simulink model "model_dyskr_z_kwantyzatorem"  (Simulink 7.5)
settings: Solver=ode45  StartTime=0.0  StopTime=5  FixedStep=0.006  MinStep=0.0006  RelTol=1e-3
undefined symbols (not defined in the file): In, J, K1, K2, Kp, Kt, lambdaN, m, Mn, psien, Rt, T, tm, Tp, Un, uz0, V, wn, Y
settings Model: Creator=Konrad  LastModifiedBy=Konrad

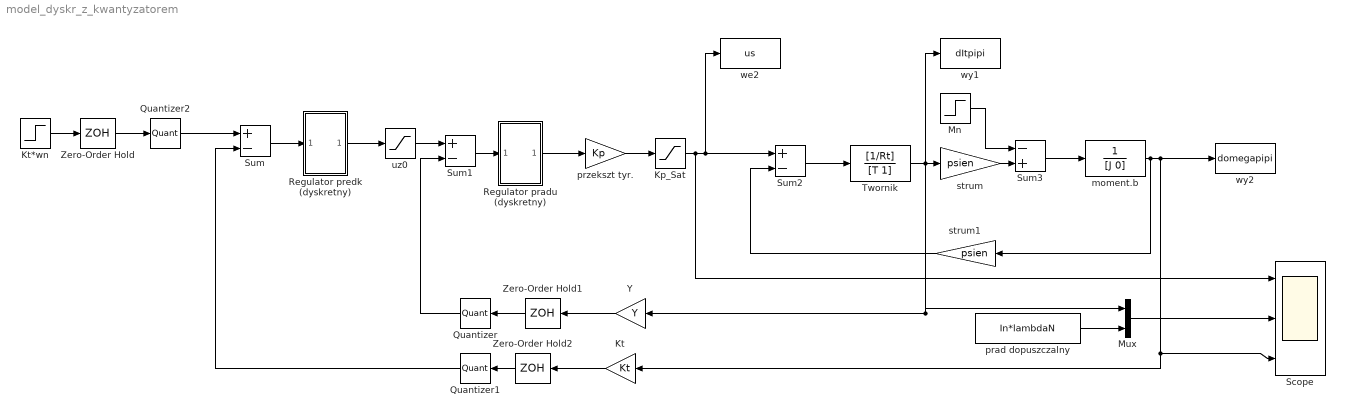
== system model_dyskr_z_kwantyzatorem ==
  Kp_Sat : Saturate  UpperLimit=1.5*Un  LowerLimit=-1.5*Un  OutDataType=fixdt(1, 16)  OutScaling=2^0
  Kt : Gain  Gain=Kt  ParameterDataType=fixdt(1, 16)  ParameterScaling=2^0  OutDataType=fixdt(1, 16)  OutScaling=2^0
  Kt*wn : Step  Time=0  After=Kt*wn  SampleTime=0
  Mn : Step  Time=tm  After=Mn  SampleTime=0
  Mux : Mux  Inputs=2
  Quantizer : Quantizer  QuantizationInterval=q  SampleTime=Tp
  Quantizer1 : Quantizer  QuantizationInterval=q  SampleTime=Tp
  Quantizer2 : Quantizer  QuantizationInterval=q  SampleTime=Tp
  Regulator pradu (dyskretny) : Subsystem  Description=Reg
  Regulator predk (dyskretny) : Subsystem  Description=Reg
  Scope : Scope  NumInputPorts=3
      settings: YMin=-5~-5~-5  YMax=5~5~5
  Sum : Sum  Inputs=+-  OutDataType=fixdt(1, 16)  OutScaling=2^-10
  Sum1 : Sum  Inputs=+-  OutDataType=fixdt(1, 16)  OutScaling=2^-10
  Sum2 : Sum  Inputs=+-  OutDataType=fixdt(1, 16)  OutScaling=2^-10
  Sum3 : Sum  Inputs=-+  OutDataType=fixdt(1, 16)  OutScaling=2^-10
  Twornik : TransferFcn  Numerator=[1/Rt]  Denominator=[T 1]
  Y : Gain  Gain=Y  ParameterDataType=fixdt(1, 16)  ParameterScaling=2^0  OutDataType=fixdt(1, 16)  OutScaling=2^0
  Zero-Order Hold : ZeroOrderHold  SampleTime=Tp
  Zero-Order Hold1 : ZeroOrderHold  SampleTime=Tp
  Zero-Order Hold2 : ZeroOrderHold  SampleTime=Tp
  moment.b : TransferFcn  Denominator=[J 0]
  prad dopuszczalny : Constant  Value=In*lambdaN  OutDataType=fixdt(1, 16)  OutScaling=2^0
  przekszt tyr. : Gain  Gain=Kp  ParameterDataType=fixdt(1, 16)  ParameterScaling=2^0  OutDataType=fixdt(1, 16)  OutScaling=2^0
  strum : Gain  Gain=psien  ParameterDataType=fixdt(1, 16)  ParameterScaling=2^0  OutDataType=fixdt(1, 16)  OutScaling=2^0
  strum1 : Gain  Gain=psien  ParameterDataType=fixdt(1, 16)  ParameterScaling=2^0  OutDataType=fixdt(1, 16)  OutScaling=2^0
  uz0 : Saturate  UpperLimit=uz0  LowerLimit=-uz0  OutDataType=fixdt(1, 16)  OutScaling=2^0
  we2 : ToWorkspace  VariableName=us  SampleTime=-1  SaveFormat=Structure
  wy1 : ToWorkspace  VariableName=dItpipi  SampleTime=-1  SaveFormat=Structure
  wy2 : ToWorkspace  VariableName=domegapipi  SampleTime=-1  SaveFormat=Structure
  wires:
  Kt*wn/1 -> Zero-Order Hold/1
  uz0/1 -> Sum1/1
  przekszt tyr./1 -> Kp_Sat/1
  Kp_Sat/1 -> Sum2/1, we2/1, Scope/1
  Sum2/1 -> Twornik/1
  Twornik/1 -> strum/1, wy1/1, Y/1, Mux/1
  moment.b/1 -> strum1/1, wy2/1, Scope/3, Kt/1
  strum/1 -> Sum3/2
  Mn/1 -> Sum3/1
  strum1/1 -> Sum2/2
  Sum3/1 -> moment.b/1
  Y/1 -> Zero-Order Hold1/1
  Kt/1 -> Zero-Order Hold2/1
  Sum/1 -> Regulator predk (dyskretny)/1(In1)
  Regulator predk (dyskretny)/1(Out1) -> uz0/1
  Sum1/1 -> Regulator pradu (dyskretny)/1(In1)
  Regulator pradu (dyskretny)/1(Out1) -> przekszt tyr./1
  prad dopuszczalny/1 -> Mux/2
  Mux/1 -> Scope/2
  Zero-Order Hold2/1 -> Quantizer1/1
  Zero-Order Hold1/1 -> Quantizer/1
  Quantizer/1 -> Sum1/2
  Quantizer1/1 -> Sum/2
  Quantizer2/1 -> Sum/1
  Zero-Order Hold/1 -> Quantizer2/1

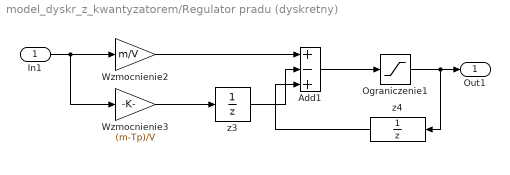
== system model_dyskr_z_kwantyzatorem/Regulator pradu (dyskretny) ==
  In1 : Inport
  Add1 : Sum  Inputs=+-+  OutDataType=fixdt(1, 16)  OutScaling=2^-10
  Ograniczenie1 : Saturate  UpperLimit=10  LowerLimit=-10  OutDataType=fixdt(1, 16)  OutScaling=2^0
  Wzmocnienie2 : Gain  Gain=m/V  ParameterDataType=fixdt(1, 16)  ParameterScaling=2^0  OutDataType=fixdt(1, 16)  OutScaling=2^0
  Wzmocnienie3 : Gain  Gain=(m-Tp)/V  ParameterDataType=fixdt(1, 16)  ParameterScaling=2^0  OutDataType=fixdt(1, 16)  OutScaling=2^0
  z3 : UnitDelay  SampleTime=-1
  z4 : UnitDelay  SampleTime=-1
  Out1 : Outport
  wires:
  In1/1 -> Wzmocnienie2/1, Wzmocnienie3/1
  Wzmocnienie2/1 -> Add1/1
  Wzmocnienie3/1 -> z3/1
  z3/1 -> Add1/2
  z4/1 -> Add1/3
  Add1/1 -> Ograniczenie1/1
  Ograniczenie1/1 -> z4/1, Out1/1

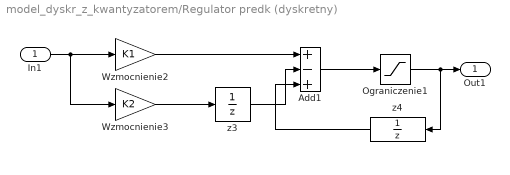
== system model_dyskr_z_kwantyzatorem/Regulator predk (dyskretny) ==
  In1 : Inport
  Add1 : Sum  Inputs=+-+  OutDataType=fixdt(1, 16)  OutScaling=2^-10
  Ograniczenie1 : Saturate  UpperLimit=10  LowerLimit=-10  OutDataType=fixdt(1, 16)  OutScaling=2^0
  Wzmocnienie2 : Gain  Gain=K1  ParameterDataType=fixdt(1, 16)  ParameterScaling=2^0  OutDataType=fixdt(1, 16)  OutScaling=2^0
  Wzmocnienie3 : Gain  Gain=K2  ParameterDataType=fixdt(1, 16)  ParameterScaling=2^0  OutDataType=fixdt(1, 16)  OutScaling=2^0
  z3 : UnitDelay  SampleTime=Tp
  z4 : UnitDelay  SampleTime=Tp
  Out1 : Outport
  wires:
  In1/1 -> Wzmocnienie2/1, Wzmocnienie3/1
  Wzmocnienie2/1 -> Add1/1
  Wzmocnienie3/1 -> z3/1
  z3/1 -> Add1/2
  z4/1 -> Add1/3
  Add1/1 -> Ograniczenie1/1
  Ograniczenie1/1 -> z4/1, Out1/1
